simulink model "DC_AGI"  (R2022b)
settings: Solver=ode4  StartTime=0.0  StopTime=tend  FixedStep=ts  RelTol=1e-3
values from neighbouring files (symbols this model uses):
  C = 80000e-6    (= 0.08)    [Parameters.m]
  C_bc_ESS = C_bc_ESS    (= 0.005)    [Parameters.m]
  C_bc_PV = C_bc_PV    (= 0.005)    [Parameters.m]
  C_bc_SC = C_bc_SC    (= 0.005)    [Parameters.m]
  C_SC_set = C_SC * Vdc_SCunit^2/Vdc_SC^2    (= 0.617283950617)    [Parameters.m]
  Cf = 0.08    [Parameters.m]
  f0 = 60    [Parameters.m]
  fc = 20    [Parameters.m]
  fc1 = 1000    [Parameters.m]
  fv = 100    [Parameters.m]
  Idcbase = Sbase/Vdc_nom    (= 1250)    [Parameters.m]
  J = [0 -1; 1 0]    [Parameters.m]
  Ki_c1 = 500    [Parameters.m]
  Ki_v = 500    [Parameters.m]
  Kp_c1 = 10    [Parameters.m]
  Kp_v = 5    [Parameters.m]
  L_bc_ESS = 4e-4    (= 0.0004)    [Parameters.m]
  L_bc_PV = 4e-4    (= 0.0004)    [Parameters.m]
  L_bc_SC = 4e-4    (= 0.0004)    [Parameters.m]
  Lf = 0.10    (= 0.1)    [Parameters.m]
  Plim_ESS = 0.4    [Parameters.m]
  Plim_PV = 0.7    [Parameters.m]
  Plim_SC = 0.3    [Parameters.m]
  Pset_ESS = 0.0    (= 0)    [Parameters.m]
  Pset_inv = Pset_PV + Pset_ESS + Pset_load    (= 0.4)    [Parameters.m]
  Pset_load = -0.1    [Parameters.m]
  Pset_PV = 0.5    [Parameters.m]
  Pset_SC = 0.0    (= 0)    [Parameters.m]
  Qset_inv = 0.0    (= 0)    [Parameters.m]
  R_bc_ESS = 1e-3    (= 0.001)    [Parameters.m]
  R_bc_PV = 1e-3    (= 0.001)    [Parameters.m]
  R_bc_SC = 1e-3    (= 0.001)    [Parameters.m]
  R_line_ESS = 1e-3    (= 0.001)    [Parameters.m]
  R_line_PV = 1e-3    (= 0.001)    [Parameters.m]
  R_line_SC = 1e-3    (= 0.001)    [Parameters.m]
  Rf = 5e-4    (= 0.0005)    [Parameters.m]
  Rg = 0.04 * 2    (= 0.08)    [Parameters.m]
  Sbase = Stotal    (= 1000000)    [Parameters.m]
  Stotal = 1e6    (= 1000000)    [Parameters.m]
  tdist1 = 2    [Parameters.m]
  tdist2 = 4    [Parameters.m]
  tESSconnect = 0.1    [Parameters.m]
  tPVconnect = 0.3    [Parameters.m]
  ts = 5e-6    (= 5e-06)    [Parameters.m]
  tSCconnect = 0.2    [Parameters.m]
  V1 = 4160    [Parameters.m]
  V2 = 400    [Parameters.m]
  Vac_peak = Vac_nom*sqrt(2)/sqrt(3)    [Parameters.m]
  Vdc_ESS = 480    [Parameters.m]
  Vdc_nom = 800    [Parameters.m]
  Vdc_PV = 480    [Parameters.m]
  Vdc_PV0 = 464.3    [Parameters.m]
  Vdc_SC = Vdc_SCunit * 180    (= 486)    [Parameters.m]
  Vdc_SC0 = Vdc_SC    (= 486)    [Parameters.m]
  Vset_inv = 1.05    [Parameters.m]
  w0 = 2*pi*f0    (= 376.991118431)    [Parameters.m]
  Zbase = Vbase^2/Sbase    (= 17.3056)    [Parameters.m]
  Zg = 0.2 * 2    (= 0.4)    [Parameters.m]
undefined symbols (not defined in the file or in its folder): Gf, Ilim, L_line_ESS, L_line_PV, Pnom, sps, Vnom
libraries: spsSeriesRLCBranchLib x12, spsControlledVoltageSourceLib x9, spsVoltageMeasurementLib x8, cstblocks x8, spsCurrentMeasurementLib x6, simulink_extras x5, spsBreakerLib x4, spsThreePhaseVIMeasurementLib x3, spsabctoAlphaBetaZeroLib x3, spsPWMGeneratorDCDCLib x3, spsTwoQuadrantDCDCConverterLib x3, spsThreePhaseSeriesRLCBranchLib x3
(part 2 of 2)

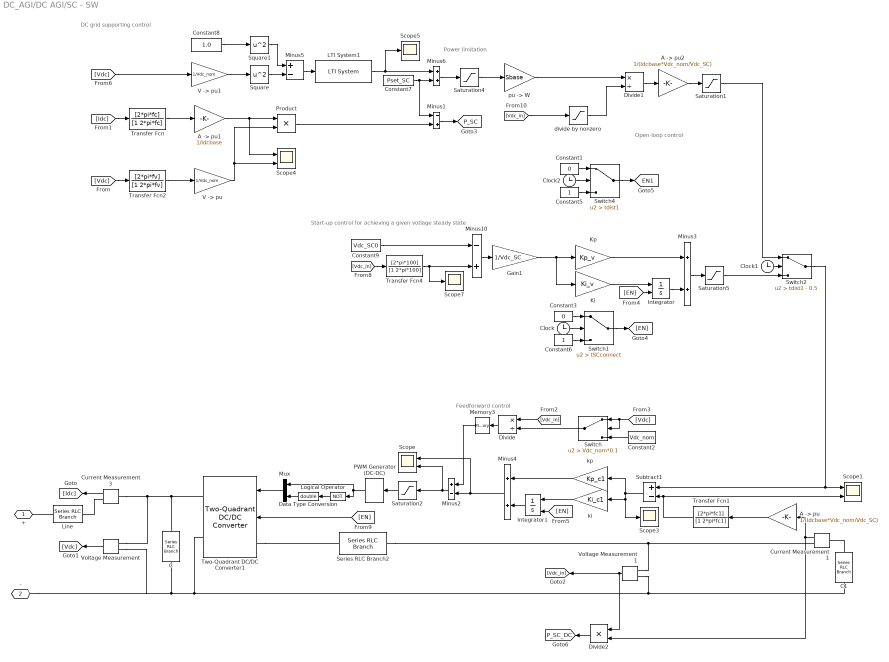
== system DC_AGI/DC AGI/SC - SW ==
  note: Open-loop control
  note: Power limitation
  note: Start-up control for achieving a given votlage steady state
  note: DC grid supporting control
  note: Feedforward control
  "A -> pu" : Gain  Gain=1/(Idcbase*Vdc_nom/Vdc_SC)
  "A -> pu1" : Gain  Gain=1/Idcbase
  "A -> pu2" : Gain  Gain=1/(Idcbase*Vdc_nom/Vdc_SC)
  C : spsSeriesRLCBranchLib/Series RLC Branch  LConnTagsString=__new0  RConnTagsString=__new0  BranchType=C  Resistance=0.001  Inductance=L_line_PV  SetiL0=off  InitialCurrent=0  Capacitance=C_bc_SC  Setx0=on  InitialVoltage=Vdc_nom  Measurements=None
  C1 : spsSeriesRLCBranchLib/Series RLC Branch  LConnTagsString=__new0  RConnTagsString=__new0  BranchType=C  Resistance=0.001  Inductance=L_line_PV  SetiL0=off  InitialCurrent=0  Capacitance=C_SC_set  Setx0=on  InitialVoltage=Vdc_SC0  Measurements=None
  Clock : Clock
  Clock1 : Clock
  Clock2 : Clock
  Constant1 : Constant  Value=0
  Constant2 : Constant  Value=Vdc_nom
  Constant3 : Constant  Value=0
  Constant5 : Constant
  Constant6 : Constant
  Constant7 : Constant  Value=Pset_SC
  Constant8 : Constant  Value=1.0
  Constant9 : Constant  Value=Vdc_SC0
  Current Measurement1 : spsCurrentMeasurementLib/Current Measurement  PhasorSimulation=off  OutputType=Complex  PSBequivalent=0
  Current Measurement3 : spsCurrentMeasurementLib/Current Measurement  PhasorSimulation=off  OutputType=Complex  PSBequivalent=0
  Data Type Conversion : DataTypeConversion  OutDataTypeStr=double  SaturateOnIntegerOverflow=off  RndMeth=Floor
  Divide : Product  Inputs=*/
  Divide1 : Product  Inputs=*/
  Divide2 : Product  Inputs=**
  Gain1 : Gain  Gain=1/Vdc_SC
  Integrator : Integrator  ExternalReset=level hold  UpperSaturationLimit=1.5  LowerSaturationLimit=-0.5
  Integrator1 : Integrator  ExternalReset=level hold  LimitOutput=on  UpperSaturationLimit=1  LowerSaturationLimit=-1
  Ki : Gain  Gain=Ki_v
  Kp : Gain  Gain=Kp_v
  LTI System1 : cstblocks/LTI System  sys=T_SC1  IC=[]
  Line : spsSeriesRLCBranchLib/Series RLC Branch  LConnTagsString=__new0  RConnTagsString=__new0  BranchType=R  Resistance=R_line_SC  Inductance=L_line_ESS  SetiL0=off  InitialCurrent=0  Capacitance=1e-6  Setx0=off  InitialVoltage=0  Measurements=None
  Logical Operator : Logic  Operator=NOT  AllPortsSameDT=off  OutDataTypeStr=boolean
  Memory3 : Memory
  Minus1 : Sum  Inputs=-+
  Minus10 : Sum  Inputs=-+
  Minus2 : Sum  Inputs=+-
  Minus3 : Sum
  Minus4 : Sum
  Minus5 : Sum  Inputs=+-
  Minus6 : Sum
  Mux : Mux  Inputs=2
  PWM Generator (DC-DC) : spsPWMGeneratorDCDCLib/PWM Generator (DC-DC)  Fsw=fw  Ts=0
  Product : Product
  Saturation1 : Saturate  UpperLimit=1.0  LowerLimit=-1.0
  Saturation2 : Saturate  UpperLimit=1  LowerLimit=0
  Saturation4 : Saturate  UpperLimit=Plim_SC  LowerLimit=-Plim_SC
  Saturation5 : Saturate  UpperLimit=1.0  LowerLimit=-1.0
  Scope : Scope  NumInputPorts=2
  Scope1 : Scope  NumInputPorts=2
  Scope3 : Scope
  Scope4 : Scope  NumInputPorts=2
  Scope5 : Scope
  Scope7 : Scope
  Series RLC Branch2 : spsSeriesRLCBranchLib/Series RLC Branch  LConnTagsString=__new0  RConnTagsString=__new0  BranchType=RL  Resistance=R_bc_SC  Inductance=L_bc_SC  SetiL0=off  InitialCurrent=Pset_SC*Idcbase*Vdc_nom/Vdc_PV  Capacitance=1e-6  Setx0=off  InitialVoltage=0  Measurements=None
  Square : Math  Operator=square
  Square1 : Math  Operator=square
  Subtract1 : Sum  Inputs=+-
  Switch : Switch  Criteria=u2 > Threshold  Threshold=Vdc_nom*0.1  SaturateOnIntegerOverflow=off  InputSameDT=off
  Switch1 : Switch  Criteria=u2 > Threshold  Threshold=tSCconnect  SaturateOnIntegerOverflow=off  InputSameDT=off
  Switch2 : Switch  Criteria=u2 > Threshold  Threshold=tdist1 - 0.5  SaturateOnIntegerOverflow=off  InputSameDT=off
  Switch4 : Switch  Criteria=u2 > Threshold  Threshold=tdist1  SaturateOnIntegerOverflow=off  InputSameDT=off
  Transfer Fcn : TransferFcn  Numerator=[2*pi*fc]  Denominator=[1 2*pi*fc]
  Transfer Fcn1 : TransferFcn  Numerator=[2*pi*fc1]  Denominator=[1 2*pi*fc1]
  Transfer Fcn2 : TransferFcn  Numerator=[2*pi*fv]  Denominator=[1 2*pi*fv]
  Transfer Fcn4 : TransferFcn  Numerator=[2*pi*100]  Denominator=[1 2*pi*100]
  Two-Quadrant DC/DC Converter1 : spsTwoQuadrantDCDCConverterLib/Two-Quadrant DC//DC Converter  ModelType=Switching devices  Ron=1e-4  Rs=1e6  Cs=inf  Vforward=[0,0]  Ron_Diode=1e-3  Rs_Diode=1e6  Cs_Diode=inf  Vf_Diode=1e-3  Rs_CurrentSource=inf  Ron_ACsource=1e-3
      settings: LibrarySourceBlock=|
      | sps_lib/Power Electronics/Two-Quadrant
      | DC//DC Converter
  "V -> pu" : Gain  Gain=1/Vdc_nom
  "V -> pu1" : Gain  Gain=1/Vdc_nom
  Voltage Measurement : spsVoltageMeasurementLib/Voltage Measurement  PhasorSimulation=off  OutputType=Complex  PSBequivalent=0
  Voltage Measurement1 : spsVoltageMeasurementLib/Voltage Measurement  PhasorSimulation=off  OutputType=Complex  PSBequivalent=0
  divide by nonzero : Saturate  UpperLimit=1e6  LowerLimit=1e-6
  ki : Gain  Gain=Ki_c1
  kp : Gain  Gain=Kp_c1
  "pu -> W" : Gain  Gain=Sbase
  + : PMIOPort  Side=Left
  - : PMIOPort  Port=2  Side=Right
  tag scope: EN1=global, P_SC=global, P_SC_DC=global
  wires:
  Constant1/1 -> Switch4/1
  Switch4/1 -> [EN1]
  Clock2/1 -> Switch4/2
  Constant5/1 -> Switch4/3
  Saturation5/1 -> Switch2/3
  Minus1/1 -> [P_SC]
  Saturation4/1 -> "pu -> W"/1
  Subtract1/1 -> ki/1, Scope3/1, kp/1
  Minus6/1 -> Saturation4/1
  Divide1/1 -> "A -> pu2"/1
  divide by nonzero/1 -> Divide1/2
  "pu -> W"/1 -> Divide1/1
  "A -> pu2"/1 -> Saturation1/1
  Clock1/1 -> Switch2/2
  Minus10/1 -> Gain1/1
  [Vdc_in] -> Transfer Fcn4/1
  Constant9/1 -> Minus10/1
  Transfer Fcn4/1 -> Minus10/2, Scope7/1
  [Idc] -> Transfer Fcn/1
  Voltage Measurement/1 -> [Vdc]
  Current Measurement3/1 -> [Idc]
  [EN] -> Two-Quadrant DC/DC Converter1/2
  Current Measurement1/1 -> Divide2/2, "A -> pu"/1
  Transfer Fcn1/1 -> Subtract1/2, Scope1/2
  Product/1 -> Minus1/2
  Switch/1 -> Divide/2
  Constant2/1 -> Switch/3
  [Vdc_in] -> Divide/1
  Divide/1 -> Memory3/1
  Voltage Measurement1/1 -> Divide2/1, [Vdc_in]
  [Vdc] -> Switch/2, Switch/1
  Minus3/1 -> Saturation5/1
  Saturation1/1 -> Switch2/1
  Ki/1 -> Integrator/1
  Integrator/1 -> Minus3/2
  Kp/1 -> Minus3/1
  kp/1 -> Minus4/1
  Integrator1/1 -> Minus4/2
  ki/1 -> Integrator1/1
  Clock/1 -> Switch1/2
  Switch1/1 -> [EN]
  Constant3/1 -> Switch1/1
  Constant6/1 -> Switch1/3
  [EN] -> Integrator/2
  [EN] -> Integrator1/2
  Constant8/1 -> Square1/1
  Square/1 -> Minus5/2
  Square1/1 -> Minus5/1
  Minus5/1 -> LTI System1/1
  Constant7/1 -> Minus6/2, Minus1/1
  LTI System1/1 -> Minus6/1, Scope5/1
  [Vdc] -> "V -> pu1"/1
  "V -> pu1"/1 -> Square/1
  "V -> pu"/1 -> Product/2, Scope4/2
  "A -> pu1"/1 -> Scope4/1, Product/1
  [Vdc] -> Transfer Fcn2/1
  Minus4/1 -> Minus2/2, Scope/1
  Gain1/1 -> Kp/1, Ki/1
  Minus2/1 -> Scope/2, Saturation2/1
  Transfer Fcn/1 -> "A -> pu1"/1
  Transfer Fcn2/1 -> "V -> pu"/1
  "A -> pu"/1 -> Transfer Fcn1/1
  Memory3/1 -> Minus2/1
  Data Type Conversion/1 -> Mux/2
  Saturation2/1 -> PWM Generator (DC-DC)/1
  PWM Generator (DC-DC)/1 -> Mux/1, Logical Operator/1
  Logical Operator/1 -> Data Type Conversion/1
  Mux/1 -> Two-Quadrant DC/DC Converter1/1
  [Vdc_in] -> divide by nonzero/1
  Divide2/1 -> [P_SC_DC]
  Switch2/1 -> Subtract1/1, Scope1/1
  connections:
  C/RConn1 -- -/RConn1 -- Voltage Measurement/LConn2 -- Two-Quadrant DC/DC Converter1/RConn2 -- C1/RConn1 -- Voltage Measurement1/LConn2
  Two-Quadrant DC/DC Converter1/LConn1 -- Series RLC Branch2/LConn1
  C1/LConn1 -- Current Measurement1/LConn1
  Series RLC Branch2/RConn1 -- Voltage Measurement1/LConn1 -- Current Measurement1/RConn1
  Current Measurement3/RConn1 -- Line/RConn1
  Current Measurement3/LConn1 -- Voltage Measurement/LConn1 -- Two-Quadrant DC/DC Converter1/RConn1 -- C/LConn1
  Line/LConn1 -- +/RConn1

== system DC_AGI/Desired (re-aggregate)/Int ==
  In : Inport
  Constant6 : Constant  Value=2*pi
  Initial : InitialCondition  Value=0
  Integrator1 : Integrator  ExternalReset=rising  InitialConditionSource=external  InitialCondition=sps.Phase_Init*pi/180  ShowStatePort=on
  Relational Operator : RelationalOperator  Operator=>  OutDataTypeStr=boolean  InputSameDT=off
  Subtract : Sum  Inputs=+-
  wt : Outport
  wires:
  Integrator1/1 -> wt/1
  Initial/1 -> Integrator1/3
  In/1 -> Integrator1/1
  Relational Operator/1 -> Integrator1/2
  Subtract/1 -> Initial/1
  Integrator1/State -> Relational Operator/1, Subtract/1
  Constant6/1 -> Relational Operator/2, Subtract/2

== system DC_AGI/Desired (re-aggregate)/Inv Tr ==
  wt : Inport
  dq : Inport  Port=2
  Fcn : Fcn  Expr=u[1]*cos(u[3]) - u[2]*sin(u[3])
  Fcn1 : Fcn  Expr=u[1]*sin(u[3]) + u[2]*cos(u[3])
  Mux : Mux  Inputs=2
  Mux2 : Mux  Inputs=[2 1]
  Mux3 : Mux  Inputs=[2 1]
  albe : Outport
  wires:
  Fcn1/1 -> Mux/2
  wt/1 -> Mux2/2, Mux3/2
  Fcn/1 -> Mux/1
  Mux/1 -> albe/1
  dq/1 -> Mux2/1, Mux3/1
  Mux2/1 -> Fcn/1
  Mux3/1 -> Fcn1/1

== system DC_AGI/Grid/Int ==
  In : Inport
  Constant6 : Constant  Value=2*pi
  Initial : InitialCondition  Value=0
  Integrator1 : Integrator  ExternalReset=rising  InitialConditionSource=external  InitialCondition=sps.Phase_Init*pi/180  ShowStatePort=on
  Relational Operator : RelationalOperator  Operator=>  OutDataTypeStr=boolean  InputSameDT=off
  Subtract : Sum  Inputs=+-
  Out : Outport
  wires:
  Integrator1/1 -> Out/1
  Initial/1 -> Integrator1/3
  In/1 -> Integrator1/1
  Relational Operator/1 -> Integrator1/2
  Subtract/1 -> Initial/1
  Integrator1/State -> Relational Operator/1, Subtract/1
  Constant6/1 -> Relational Operator/2, Subtract/2

== system DC_AGI/Grid (the same)/Int ==
  In : Inport
  Constant6 : Constant  Value=2*pi
  Initial : InitialCondition  Value=0
  Integrator1 : Integrator  ExternalReset=rising  InitialConditionSource=external  InitialCondition=sps.Phase_Init*pi/180  ShowStatePort=on
  Relational Operator : RelationalOperator  Operator=>  OutDataTypeStr=boolean  InputSameDT=off
  Subtract : Sum  Inputs=+-
  Out : Outport
  wires:
  Integrator1/1 -> Out/1
  Initial/1 -> Integrator1/3
  In/1 -> Integrator1/1
  Relational Operator/1 -> Integrator1/2
  Subtract/1 -> Initial/1
  Integrator1/State -> Relational Operator/1, Subtract/1
  Constant6/1 -> Relational Operator/2, Subtract/2

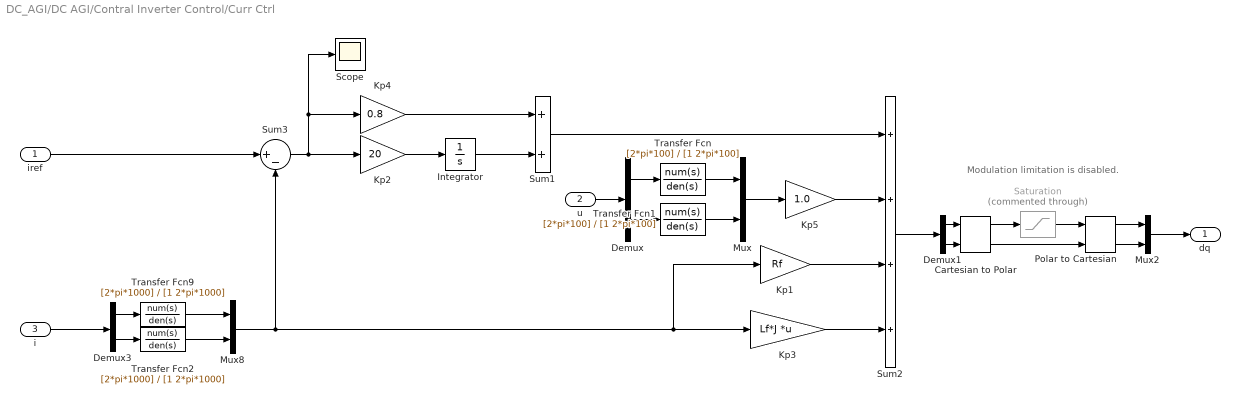
== system DC_AGI/DC AGI/Contral Inverter Control/Curr Ctrl ==
  note: Modulation limitation is disabled.
  iref : Inport
  "u " : Inport  Port=2
  i : Inport  Port=3
  Cartesian to Polar : simulink_extras/Transformations/Cartesian to Polar
  Demux : Demux  Outputs=2
  Demux1 : Demux  Outputs=2
  Demux3 : Demux  Outputs=2
  Integrator : Integrator  InitialCondition=[1 0]
  Kp1 : Gain  Gain=Rf  SaturateOnIntegerOverflow=on  OutDataTypeStr=Inherit: Same as input  ParamDataTypeStr=Inherit: Same as input
  Kp2 : Gain  Gain=20  SaturateOnIntegerOverflow=on  OutDataTypeStr=Inherit: Same as input  ParamDataTypeStr=Inherit: Same as input
  Kp3 : Gain  Gain=Lf*J  Multiplication=Matrix(K*u)  SaturateOnIntegerOverflow=on  OutDataTypeStr=Inherit: Same as input  ParamDataTypeStr=Inherit: Same as input
  Kp4 : Gain  Gain=0.8  SaturateOnIntegerOverflow=on  OutDataTypeStr=Inherit: Same as input  ParamDataTypeStr=Inherit: Same as input
  Kp5 : Gain  Gain=1.0  SaturateOnIntegerOverflow=on  OutDataTypeStr=Inherit: Same as input  ParamDataTypeStr=Inherit: Same as input
  Mux : Mux  Inputs=2
  Mux2 : Mux  Inputs=2
  Mux8 : Mux  Inputs=2
  Polar to Cartesian : simulink_extras/Transformations/Polar to Cartesian
  Saturation : Saturate  Commented=through  UpperLimit=1.5  LowerLimit=0
  Scope : Scope
  Sum1 : Sum
  Sum2 : Sum  Inputs=++++
  Sum3 : Sum  Inputs=|+-
  Transfer Fcn : TransferFcn  Numerator=[2*pi*100]  Denominator=[1 2*pi*100]
  Transfer Fcn1 : TransferFcn  Numerator=[2*pi*100]  Denominator=[1 2*pi*100]
  Transfer Fcn2 : TransferFcn  Numerator=[2*pi*1000]  Denominator=[1 2*pi*1000]
  Transfer Fcn9 : TransferFcn  Numerator=[2*pi*1000]  Denominator=[1 2*pi*1000]
  dq : Outport
  wires:
  Demux3/2 -> Transfer Fcn2/1
  i/1 -> Demux3/1
  Demux3/1 -> Transfer Fcn9/1
  Transfer Fcn9/1 -> Mux8/1
  Transfer Fcn2/1 -> Mux8/2
  iref/1 -> Sum3/1
  Saturation/1 -> Polar to Cartesian/1
  Polar to Cartesian/1 -> Mux2/1
  Sum2/1 -> Demux1/1
  Demux1/1 -> Cartesian to Polar/1
  Cartesian to Polar/1 -> Saturation/1
  Cartesian to Polar/2 -> Polar to Cartesian/2
  Polar to Cartesian/2 -> Mux2/2
  Demux1/2 -> Cartesian to Polar/2
  Transfer Fcn/1 -> Mux/1
  Transfer Fcn1/1 -> Mux/2
  Demux/2 -> Transfer Fcn1/1
  Demux/1 -> Transfer Fcn/1
  Mux/1 -> Kp5/1
  Kp5/1 -> Sum2/2
  "u "/1 -> Demux/1
  Kp3/1 -> Sum2/4
  Kp1/1 -> Sum2/3
  Mux2/1 -> dq/1
  Kp2/1 -> Integrator/1
  Mux8/1 -> Kp3/1, Kp1/1, Sum3/2
  Integrator/1 -> Sum1/2
  Kp4/1 -> Sum1/1
  Sum3/1 -> Kp2/1, Kp4/1, Scope/1
  Sum1/1 -> Sum2/1

== system DC_AGI/DC AGI/Contral Inverter Control/Curr T ==
  abc : Inport
  In2 : Inport  Port=2
  Demux : Demux  Outputs=3
  Mux1 : Mux  Inputs=2
  Subsystem : Subsystem
  Terminator2 : Terminator
  abc to Alpha-Beta-Zero : spsabctoAlphaBetaZeroLib/abc to Alpha-Beta-Zero
  dq : Outport
  wires:
  In2/1 -> Subsystem/2(wt)
  Mux1/1 -> Subsystem/1(albe)
  abc/1 -> abc to Alpha-Beta-Zero/1
  Demux/2 -> Mux1/2
  Demux/1 -> Mux1/1
  Demux/3 -> Terminator2/1
  abc to Alpha-Beta-Zero/1 -> Demux/1
  Subsystem/1(dq) -> dq/1

== system DC_AGI/DC AGI/Contral Inverter Control/Curr in T ==
  abc : Inport
  In2 : Inport  Port=2
  Demux : Demux  Outputs=3
  Mux1 : Mux  Inputs=2
  Subsystem : Subsystem
  Terminator2 : Terminator
  abc to Alpha-Beta-Zero : spsabctoAlphaBetaZeroLib/abc to Alpha-Beta-Zero
  dq : Outport
  wires:
  Subsystem/1(dq) -> dq/1
  In2/1 -> Subsystem/2(wt)
  Mux1/1 -> Subsystem/1(albe)
  abc/1 -> abc to Alpha-Beta-Zero/1
  Demux/2 -> Mux1/2
  Demux/1 -> Mux1/1
  Demux/3 -> Terminator2/1
  abc to Alpha-Beta-Zero/1 -> Demux/1

== system DC_AGI/DC AGI/Contral Inverter Control/Int ==
  In : Inport
  Constant6 : Constant  Value=2*pi
  Initial : InitialCondition  Value=0
  Integrator1 : Integrator  ExternalReset=rising  InitialConditionSource=external  InitialCondition=sps.Phase_Init*pi/180  ShowStatePort=on
  Relational Operator : RelationalOperator  Operator=>  OutDataTypeStr=boolean  InputSameDT=off
  Subtract : Sum  Inputs=+-
  Out : Outport
  wires:
  Integrator1/1 -> Out/1
  Initial/1 -> Integrator1/3
  In/1 -> Integrator1/1
  Relational Operator/1 -> Integrator1/2
  Subtract/1 -> Initial/1
  Integrator1/State -> Relational Operator/1, Subtract/1
  Constant6/1 -> Relational Operator/2, Subtract/2

== system DC_AGI/DC AGI/Contral Inverter Control/Inv Tr ==
  dq : Inport
  wt : Inport  Port=2
  Fcn : Fcn  Expr=u[1]*cos(u[3]) - u[2]*sin(u[3])
  Fcn1 : Fcn  Expr=u[1]*sin(u[3]) + u[2]*cos(u[3])
  Mux : Mux  Inputs=2
  Mux2 : Mux  Inputs=[2 1]
  Mux3 : Mux  Inputs=[2 1]
  albe : Outport
  wires:
  Fcn1/1 -> Mux/2
  wt/1 -> Mux2/2, Mux3/2
  Fcn/1 -> Mux/1
  Mux/1 -> albe/1
  dq/1 -> Mux2/1, Mux3/1
  Mux2/1 -> Fcn/1
  Mux3/1 -> Fcn1/1

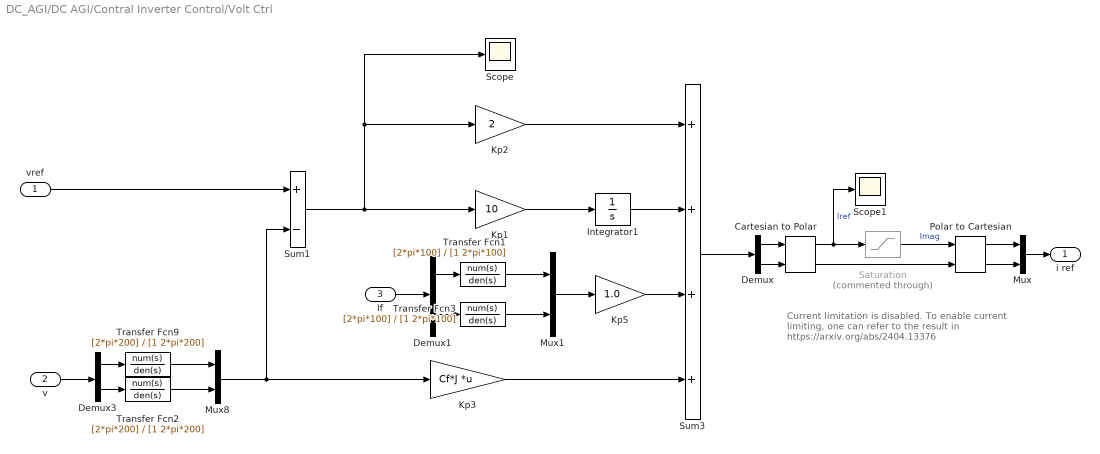
== system DC_AGI/DC AGI/Contral Inverter Control/Volt Ctrl ==
  note: Current limitation is disabled.
      | To enable current limiting, one can
      | refer to the result in https://arxiv.org/abs/2404.13376
  vref : Inport
  v : Inport  Port=2
  If : Inport  Port=3
  Cartesian to Polar : simulink_extras/Transformations/Cartesian to Polar
  Demux : Demux  Outputs=2
  Demux1 : Demux  Outputs=2
  Demux3 : Demux  Outputs=2
  Integrator1 : Integrator  InitialCondition=[0 0]
  Kp1 : Gain  Gain=10  SaturateOnIntegerOverflow=on  OutDataTypeStr=Inherit: Same as input  ParamDataTypeStr=Inherit: Same as input
  Kp2 : Gain  Gain=2  SaturateOnIntegerOverflow=on  OutDataTypeStr=Inherit: Same as input  ParamDataTypeStr=Inherit: Same as input
  Kp3 : Gain  Gain=Cf*J  Multiplication=Matrix(K*u)  SaturateOnIntegerOverflow=on  OutDataTypeStr=Inherit: Same as input  ParamDataTypeStr=Inherit: Same as input
  Kp5 : Gain  Gain=1.0  SaturateOnIntegerOverflow=on  OutDataTypeStr=Inherit: Same as input  ParamDataTypeStr=Inherit: Same as input
  Mux : Mux  Inputs=2
  Mux1 : Mux  Inputs=2
  Mux8 : Mux  Inputs=2
  Polar to Cartesian : simulink_extras/Transformations/Polar to Cartesian
  Saturation : Saturate  Commented=through  UpperLimit=Ilim  LowerLimit=0
  Scope : Scope
  Scope1 : Scope
  Sum1 : Sum  Inputs=+-
  Sum3 : Sum  Inputs=++++
  Transfer Fcn1 : TransferFcn  Numerator=[2*pi*100]  Denominator=[1 2*pi*100]
  Transfer Fcn2 : TransferFcn  Numerator=[2*pi*200]  Denominator=[1 2*pi*200]
  Transfer Fcn3 : TransferFcn  Numerator=[2*pi*100]  Denominator=[1 2*pi*100]
  Transfer Fcn9 : TransferFcn  Numerator=[2*pi*200]  Denominator=[1 2*pi*200]
  i ref : Outport
  wires:
  vref/1 -> Sum1/1
  Demux1/2 -> Transfer Fcn3/1
  Demux/1 -> Cartesian to Polar/1
  Mux8/1 -> Kp3/1, Sum1/2
  Cartesian to Polar/2 -> Polar to Cartesian/2
  Demux/2 -> Cartesian to Polar/2
  Saturation/1 -> Polar to Cartesian/1  "Imag"
  Integrator1/1 -> Sum3/2
  Mux1/1 -> Kp5/1
  Kp1/1 -> Integrator1/1
  Transfer Fcn1/1 -> Mux1/1
  Kp2/1 -> Sum3/1
  Transfer Fcn3/1 -> Mux1/2
  If/1 -> Demux1/1
  Demux1/1 -> Transfer Fcn1/1
  Kp5/1 -> Sum3/3
  Sum3/1 -> Demux/1
  Sum1/1 -> Kp2/1, Scope/1, Kp1/1
  Polar to Cartesian/1 -> Mux/1
  Polar to Cartesian/2 -> Mux/2
  Mux/1 -> i ref/1
  Cartesian to Polar/1 -> Saturation/1, Scope1/1  "Iref"
  Transfer Fcn2/1 -> Mux8/2
  Transfer Fcn9/1 -> Mux8/1
  Demux3/2 -> Transfer Fcn2/1
  Demux3/1 -> Transfer Fcn9/1
  v/1 -> Demux3/1
  Kp3/1 -> Sum3/4

== system DC_AGI/DC AGI/Contral Inverter Control/Volt T ==
  abc : Inport
  In2 : Inport  Port=2
  Demux : Demux  Outputs=3
  Mux1 : Mux  Inputs=2
  Subsystem : Subsystem
  Terminator2 : Terminator
  abc to Alpha-Beta-Zero : spsabctoAlphaBetaZeroLib/abc to Alpha-Beta-Zero
  dq : Outport
  wires:
  Subsystem/1(dq) -> dq/1
  abc to Alpha-Beta-Zero/1 -> Demux/1
  Demux/3 -> Terminator2/1
  Demux/1 -> Mux1/1
  Demux/2 -> Mux1/2
  abc/1 -> abc to Alpha-Beta-Zero/1
  Mux1/1 -> Subsystem/1(albe)
  In2/1 -> Subsystem/2(wt)

== system DC_AGI/DC AGI/Contral Inverter Control/Curr T/Subsystem ==
  note: d = al*cos(wt) + be*sin(wt)
  note: q = -al*sin(wt) + be*cos(wt)
  albe : Inport
  wt : Inport  Port=2
  Fcn : Fcn  Expr=u[1]*cos(u[3]) + u[2]*sin(u[3])
  Fcn1 : Fcn  Expr=-u[1]*sin(u[3]) + u[2]*cos(u[3])
  Mux : Mux  Inputs=2
  Mux2 : Mux  Inputs=[2 1]
  Mux3 : Mux  Inputs=[2 1]
  dq : Outport
  wires:
  Fcn1/1 -> Mux/2
  wt/1 -> Mux2/2, Mux3/2
  Fcn/1 -> Mux/1
  Mux/1 -> dq/1
  albe/1 -> Mux2/1, Mux3/1
  Mux2/1 -> Fcn/1
  Mux3/1 -> Fcn1/1

== system DC_AGI/DC AGI/Contral Inverter Control/Curr in T/Subsystem ==
  note: d = al*cos(wt) + be*sin(wt)
  note: q = -al*sin(wt) + be*cos(wt)
  albe : Inport
  wt : Inport  Port=2
  Fcn : Fcn  Expr=u[1]*cos(u[3]) + u[2]*sin(u[3])
  Fcn1 : Fcn  Expr=-u[1]*sin(u[3]) + u[2]*cos(u[3])
  Mux : Mux  Inputs=2
  Mux2 : Mux  Inputs=[2 1]
  Mux3 : Mux  Inputs=[2 1]
  dq : Outport
  wires:
  Fcn1/1 -> Mux/2
  wt/1 -> Mux2/2, Mux3/2
  Fcn/1 -> Mux/1
  Mux/1 -> dq/1
  albe/1 -> Mux2/1, Mux3/1
  Mux2/1 -> Fcn/1
  Mux3/1 -> Fcn1/1

== system DC_AGI/DC AGI/Contral Inverter Control/Volt T/Subsystem ==
  note: q = -al*sin(wt) + be*cos(wt)
  note: d = al*cos(wt) + be*sin(wt)
  albe : Inport
  wt : Inport  Port=2
  Fcn : Fcn  Expr=u[1]*cos(u[3]) + u[2]*sin(u[3])
  Fcn1 : Fcn  Expr=-u[1]*sin(u[3]) + u[2]*cos(u[3])
  Mux : Mux  Inputs=2
  Mux2 : Mux  Inputs=[2 1]
  Mux3 : Mux  Inputs=[2 1]
  dq : Outport
  wires:
  Mux3/1 -> Fcn1/1
  Mux2/1 -> Fcn/1
  albe/1 -> Mux3/1, Mux2/1
  Mux/1 -> dq/1
  Fcn/1 -> Mux/1
  wt/1 -> Mux3/2, Mux2/2
  Fcn1/1 -> Mux/2
